simulink model "StateMachineModelFromFiles"  (R2021b)
settings: Solver=VariableStepAuto  StartTime=0.0  StopTime=inf  RelTol=1e-3
model workspace (MATLAB code in the model file):
  | % Add the class folders into the path.
  | addpath model
  | addpath utils
  | 
  | %% Loading data from files.
  | % Data for supervisor 1.
  | utils = StateMachineUtils;
  | 
  | % From TCT: Load all events' number.
  | utils = utils.loadEventsInAds('resources/tct/ALLEVENT.ADS');
  | 
  | % From TCT: Disabled events in each state.
  | utils = utils.loadDisabledEventsInPdt('resources/tct/supervisor1/DATA_SIMSUP1_MG1.PDT');
  | 
  | % From TCT: Transition matrix.
  | utils = utils.loadTransitionsInAds('resources/tct/supervisor1/SIMSUP1_MG1.ADS');
  | 
  | % Parameters for the block.
  | encodedStates1 = StateEncoder.encode(utils.statesArray);
  | 
  | transitions1 = utils.transitions;
  | 
  | allEvents1 = utils.eventsArray;
  | 
  | % Data for supervisor 2.
  | utils2 = StateMachineUtils;
  | 
  | % From TCT: Load all events' number.
  | utils2 = utils2.loadEventsInAds('resources/tct/ALLEVENT.ADS');
  | 
  | % From TCT: Disabled events in each state.
  | utils2 = utils2.loadDisabledEventsInPdt('resources/tct/supervisor2/DATA_SIMSUP2_MG1.PDT');
  | 
  | % From TCT: Transition matrix.
  | utils2 = utils2.loadTransitionsInAds('resources/tct/supervisor2/SIMSUP2_MG1.ADS');
  | 
  | % Parameters for the block.
  | encodedStates2 = StateEncoder.encode(utils2.statesArray);
  | 
  | transitions2 = utils2.transitions;
  | 
  | allEvents2 = utils2.eventsArray;
  | 
  | 
  | % Data for supervisor 3.
  | utils3 = StateMachineUtils;
  | 
  | % From TCT: Load all events' number.
  | utils3 = utils3.loadEventsInAds('resources/tct/ALLEVENT.ADS');
  | 
  | % From TCT: Disabled events in each state.
  | utils3 = utils3.loadDisabledEventsInPdt('resources/tct/supervisor3/DATA_SIMSUP3_MG1.PDT');
  | 
  | % From TCT: Transition matrix.
  | utils3 = utils3.loadTransitionsInAds('resources/tct/supervisor3/SIMSUP3_MG1.ADS');
  | 
  | % Parameters for the block.
  | encodedStates3 = StateEncoder.encode(utils3.statesArray);
  | 
  | transitions3 = utils3.transitions;
  | 
  | allEvents3 = utils3.eventsArray;
settings Model: Creator=andrerangel  LastModifiedBy=andrerangel

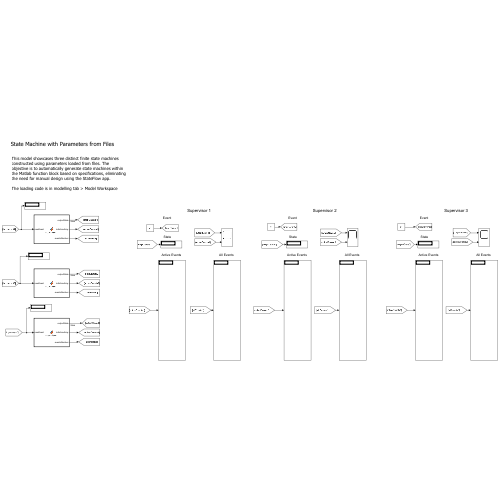
[thumbnail: Simulink's stored preview of the top-level diagram]
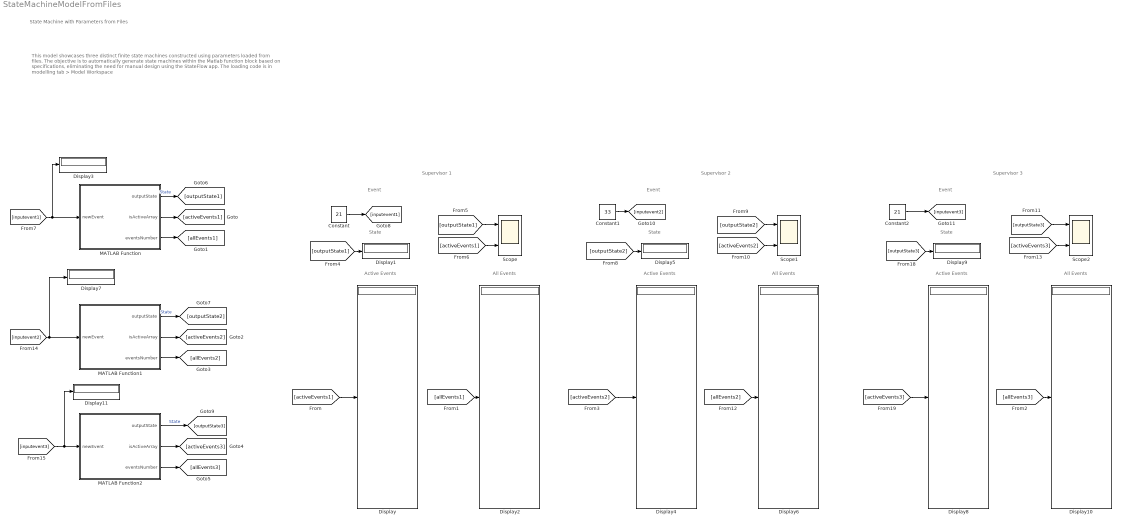
== system StateMachineModelFromFiles ==
  note: This model showcases three distinct finite state machines constructed using parameters loaded from files. The objective is to automatically generate state machines within the Matlab function block based on specifications, eliminating the need for manual design using the StateFlow app.
      |
      | The loading code is in modelling tab > Model Workspace
  note: State Machine with Parameters from Files
  note: Active Events
  note: State
  note: Event
  note: Supervisor 1
  note: All Events
  note: All Events
  note: Supervisor 2
  note: Active Events
  note: State
  note: Event
  note: Active Events
  note: State
  note: Event
  note: Supervisor 3
  note: All Events
  Constant : Constant  Value=21
  Constant1 : Constant  Value=33
  Constant2 : Constant  Value=21
  Display{,1..11} (12 alike) : Display
  MATLAB Function : MATLAB Function  TreatAsAtomicUnit=on
  MATLAB Function1 : MATLAB Function  TreatAsAtomicUnit=on
  MATLAB Function2 : MATLAB Function  TreatAsAtomicUnit=on
  Scope : Scope  NumInputPorts=2
  Scope1 : Scope  NumInputPorts=2
  Scope2 : Scope  NumInputPorts=2
  wires:
  Constant1/1 -> [inputevent2]
  MATLAB Function/2(isActiveArray) -> [activeEvents1]
  [activeEvents1] -> Display/1
  MATLAB Function/3(eventsNumber) -> [allEvents1]
  [allEvents1] -> Display2/1
  MATLAB Function1/2(isActiveArray) -> [activeEvents2]
  MATLAB Function1/3(eventsNumber) -> [allEvents2]
  MATLAB Function2/3(eventsNumber) -> [allEvents3]
  MATLAB Function2/2(isActiveArray) -> [activeEvents3]
  Constant2/1 -> [inputevent3]
  MATLAB Function/1(outputState) -> [outputState1]  "State"
  [outputState1] -> Display1/1
  [outputState1] -> Scope/1
  MATLAB Function1/1(outputState) -> [outputState2]  "State"
  [activeEvents1] -> Scope/2
  [inputevent1] -> Display3/1, MATLAB Function/1(newEvent)
  [activeEvents2] -> Scope1/2
  [activeEvents2] -> Display4/1
  [allEvents2] -> Display6/1
  [outputState2] -> Display5/1
  [inputevent2] -> MATLAB Function1/1(newEvent), Display7/1
  [outputState2] -> Scope1/1
  [inputevent3] -> MATLAB Function2/1(newEvent), Display11/1
  [activeEvents3] -> Scope2/2
  [outputState3] -> Scope2/1
  [outputState3] -> Display9/1
  [allEvents3] -> Display10/1
  [activeEvents3] -> Display8/1
  MATLAB Function2/1(outputState) -> [outputState3]  "State"
  Constant/1 -> [inputevent1]

== matlab function StateMachineModelFromFiles/MATLAB Function1 ==
  data: newEvent input; outputState output size=[1 1]; isActiveArray output; eventsNumber output; allEvents2 parameter; transitions2 parameter; encodedStates2 parameter
function [outputState, isActiveArray, eventsNumber] = supervisor1(newEvent, allEvents2, transitions2, encodedStates2)
% State Machine with parameters from files.

% Initialize a persistent object. Its value will not be erased as this
% block finishes.
persistent stateMachine

% Assign the persistent object to the StateMachine class with data passed
% as parameters.
if (isempty(stateMachine))
    statesArray = StateEncoder.decode(encodedStates2);                        
    stateMachine = StateMachine(statesArray, transitions2, allEvents2);
end

stateMachine.inputEvent = newEvent;
outputState = stateMachine.currentState.number;
isActiveArray = stateMachine.currentState.activeEvents;
eventsNumber = stateMachine.eventsArray;

== matlab function StateMachineModelFromFiles/MATLAB Function ==
  data: newEvent input; outputState output size=[1 1]; isActiveArray output; eventsNumber output; allEvents1 parameter; transitions1 parameter; encodedStates1 parameter
function [outputState, isActiveArray, eventsNumber] = supervisor1(newEvent, allEvents1, transitions1, encodedStates1)
% State Machine with parameters from files.

% Initialize a persistent object. Its value will not be erased as this
% block finishes.
persistent stateMachine

% Assign the persistent object to the StateMachine class with data passed
% as parameters.
if (isempty(stateMachine))
    statesArray = StateEncoder.decode(encodedStates1);                        
    stateMachine = StateMachine(statesArray, transitions1, allEvents1);
end

stateMachine.inputEvent = newEvent;
outputState = stateMachine.currentState.number;
isActiveArray = stateMachine.currentState.activeEvents;
eventsNumber = stateMachine.eventsArray;

== matlab function StateMachineModelFromFiles/MATLAB Function2 ==
  data: newEvent input; outputState output size=[1 1]; isActiveArray output; eventsNumber output; allEvents3 parameter; transitions3 parameter; encodedStates3 parameter
function [outputState, isActiveArray, eventsNumber] = supervisor1(newEvent, allEvents3, transitions3, encodedStates3)
% State Machine with parameters from files.

% Initialize a persistent object. Its value will not be erased as this
% block finishes.
persistent stateMachine

% Assign the persistent object to the StateMachine class with data passed
% as parameters.
if (isempty(stateMachine))
    statesArray = StateEncoder.decode(encodedStates3);                        
    stateMachine = StateMachine(statesArray, transitions3, allEvents3);
end

stateMachine.inputEvent = newEvent;
outputState = stateMachine.currentState.number;
isActiveArray = stateMachine.currentState.activeEvents;
eventsNumber = stateMachine.eventsArray;
